simulink model "px4_6dof_quadrotor_bus"  (R2021b)
settings: Solver=VariableStepAuto  StartTime=0.0  StopTime=10.0  FixedStep=plant.motor.dynamic_time_sample/10  RelTol=1e-3
undefined symbols (not defined in the file or in its folder): angular_rate, ax, ay, az, body, controller, DiscIntNeverNeededParam, dphi, dpsi, dtheta, lag, land_detector, lead, magnitude, ned, notch, phi, pitch, plant, psi, rad, roll, s, theta, thrust, vx, vy, vz, w1, w2, w3, w4, x, y, yaw, z
libraries: cstblocks x33, aerolibconvert2 x4, simulink_extras x3, simulink x3, sharedtransform x1
(part 2 of 2)

== system px4_6dof_quadrotor_bus/plant/control2motors/Plant1/Subsystem ==
  In1 : Inport
  Discrete-Time Integrator : DiscreteIntegrator  SampleTime=-1  ICPrevOutput=DiscIntNeverNeededParam  ICPrevScaledInput=DiscIntNeverNeededParam
  Gain : Gain  Gain=plant.motor.r
  Gain1 : Gain  Gain=1/plant.motor.l
  Sum : Sum  Inputs=|+-
  Im : Outport
  wires:
  Gain/1 -> Sum/2
  Gain1/1 -> Discrete-Time Integrator/1
  Discrete-Time Integrator/1 -> Im/1, Gain/1
  Sum/1 -> Gain1/1
  In1/1 -> Sum/1

== system px4_6dof_quadrotor_bus/plant/control2motors/Plant1/Subsystem1 ==
  In1 : Inport
  Discrete-Time Integrator : DiscreteIntegrator  SampleTime=plant.motor.electric_time_sample  ICPrevOutput=DiscIntNeverNeededParam  ICPrevScaledInput=DiscIntNeverNeededParam
  Gain : Gain  Gain=1/plant.motor.j_m
  Out1 : Outport
  wires:
  Gain/1 -> Out1/1
  Discrete-Time Integrator/1 -> Gain/1
  In1/1 -> Discrete-Time Integrator/1

== system px4_6dof_quadrotor_bus/plant/control2motors/Plant1/Subsystem2 ==
  In1 : Inport
  Discrete-Time Integrator : DiscreteIntegrator  SampleTime=plant.motor.electric_time_sample  ICPrevOutput=DiscIntNeverNeededParam  ICPrevScaledInput=DiscIntNeverNeededParam
  Gain : Gain  Gain=1/plant.motor.j_l
  Out1 : Outport
  wires:
  Gain/1 -> Out1/1
  In1/1 -> Discrete-Time Integrator/1
  Discrete-Time Integrator/1 -> Gain/1

== system px4_6dof_quadrotor_bus/plant/control2motors/Plant1/Subsystem3 ==
  dvel : Inport
  Add : Sum
  Discrete-Time Integrator : DiscreteIntegrator  SampleTime=plant.motor.electric_time_sample  ICPrevOutput=DiscIntNeverNeededParam  ICPrevScaledInput=DiscIntNeverNeededParam
  Gain2 : Gain  Gain=plant.motor.k_v
  Gain5 : Gain  Gain=plant.motor.k_k
  Tload : Outport
  wires:
  Add/1 -> Tload/1
  Gain2/1 -> Add/1
  Gain5/1 -> Add/2
  dvel/1 -> Discrete-Time Integrator/1, Gain2/1
  Discrete-Time Integrator/1 -> Gain5/1

== system px4_6dof_quadrotor_bus/plant/control2motors/Plant2/Subsystem ==
  In1 : Inport
  Discrete-Time Integrator : DiscreteIntegrator  SampleTime=-1  ICPrevOutput=DiscIntNeverNeededParam  ICPrevScaledInput=DiscIntNeverNeededParam
  Gain : Gain  Gain=plant.motor.r
  Gain1 : Gain  Gain=1/plant.motor.l
  Sum : Sum  Inputs=|+-
  Im : Outport
  wires:
  Gain/1 -> Sum/2
  Gain1/1 -> Discrete-Time Integrator/1
  Discrete-Time Integrator/1 -> Im/1, Gain/1
  Sum/1 -> Gain1/1
  In1/1 -> Sum/1

== system px4_6dof_quadrotor_bus/plant/control2motors/Plant2/Subsystem1 ==
  In1 : Inport
  Discrete-Time Integrator : DiscreteIntegrator  SampleTime=plant.motor.electric_time_sample  ICPrevOutput=DiscIntNeverNeededParam  ICPrevScaledInput=DiscIntNeverNeededParam
  Gain : Gain  Gain=1/plant.motor.j_m
  Out1 : Outport
  wires:
  Gain/1 -> Out1/1
  Discrete-Time Integrator/1 -> Gain/1
  In1/1 -> Discrete-Time Integrator/1

== system px4_6dof_quadrotor_bus/plant/control2motors/Plant2/Subsystem2 ==
  In1 : Inport
  Discrete-Time Integrator : DiscreteIntegrator  SampleTime=plant.motor.electric_time_sample  ICPrevOutput=DiscIntNeverNeededParam  ICPrevScaledInput=DiscIntNeverNeededParam
  Gain : Gain  Gain=1/plant.motor.j_l
  Out1 : Outport
  wires:
  Gain/1 -> Out1/1
  In1/1 -> Discrete-Time Integrator/1
  Discrete-Time Integrator/1 -> Gain/1

== system px4_6dof_quadrotor_bus/plant/control2motors/Plant2/Subsystem3 ==
  dvel : Inport
  Add : Sum
  Discrete-Time Integrator : DiscreteIntegrator  SampleTime=plant.motor.electric_time_sample  ICPrevOutput=DiscIntNeverNeededParam  ICPrevScaledInput=DiscIntNeverNeededParam
  Gain2 : Gain  Gain=plant.motor.k_v
  Gain5 : Gain  Gain=plant.motor.k_k
  Tload : Outport
  wires:
  Add/1 -> Tload/1
  Gain2/1 -> Add/1
  Gain5/1 -> Add/2
  dvel/1 -> Discrete-Time Integrator/1, Gain2/1
  Discrete-Time Integrator/1 -> Gain5/1

== system px4_6dof_quadrotor_bus/plant/control2motors/Plant3/Subsystem ==
  In1 : Inport
  Discrete-Time Integrator : DiscreteIntegrator  SampleTime=-1  ICPrevOutput=DiscIntNeverNeededParam  ICPrevScaledInput=DiscIntNeverNeededParam
  Gain : Gain  Gain=plant.motor.r
  Gain1 : Gain  Gain=1/plant.motor.l
  Sum : Sum  Inputs=|+-
  Im : Outport
  wires:
  Gain/1 -> Sum/2
  Gain1/1 -> Discrete-Time Integrator/1
  Discrete-Time Integrator/1 -> Im/1, Gain/1
  Sum/1 -> Gain1/1
  In1/1 -> Sum/1

== system px4_6dof_quadrotor_bus/plant/control2motors/Plant3/Subsystem1 ==
  In1 : Inport
  Discrete-Time Integrator : DiscreteIntegrator  SampleTime=plant.motor.electric_time_sample  ICPrevOutput=DiscIntNeverNeededParam  ICPrevScaledInput=DiscIntNeverNeededParam
  Gain : Gain  Gain=1/plant.motor.j_m
  Out1 : Outport
  wires:
  Gain/1 -> Out1/1
  Discrete-Time Integrator/1 -> Gain/1
  In1/1 -> Discrete-Time Integrator/1

== system px4_6dof_quadrotor_bus/plant/control2motors/Plant3/Subsystem2 ==
  In1 : Inport
  Discrete-Time Integrator : DiscreteIntegrator  SampleTime=plant.motor.electric_time_sample  ICPrevOutput=DiscIntNeverNeededParam  ICPrevScaledInput=DiscIntNeverNeededParam
  Gain : Gain  Gain=1/plant.motor.j_l
  Out1 : Outport
  wires:
  Gain/1 -> Out1/1
  In1/1 -> Discrete-Time Integrator/1
  Discrete-Time Integrator/1 -> Gain/1

== system px4_6dof_quadrotor_bus/plant/control2motors/Plant3/Subsystem3 ==
  dvel : Inport
  Add : Sum
  Discrete-Time Integrator : DiscreteIntegrator  SampleTime=plant.motor.electric_time_sample  ICPrevOutput=DiscIntNeverNeededParam  ICPrevScaledInput=DiscIntNeverNeededParam
  Gain2 : Gain  Gain=plant.motor.k_v
  Gain5 : Gain  Gain=plant.motor.k_k
  Tload : Outport
  wires:
  Add/1 -> Tload/1
  Gain2/1 -> Add/1
  Gain5/1 -> Add/2
  dvel/1 -> Discrete-Time Integrator/1, Gain2/1
  Discrete-Time Integrator/1 -> Gain5/1

== system px4_6dof_quadrotor_bus/plant/control2motors/Velocity Controller/Lag1 ==
  In1 : Inport
  LTI System : cstblocks/LTI System  sys=lag(Freq,Beta)  IC=[]
  Out1 : Outport
  wires:
  In1/1 -> LTI System/1
  LTI System/1 -> Out1/1

== system px4_6dof_quadrotor_bus/plant/control2motors/Velocity Controller/Notch ==
  In1 : Inport
  LTI System : cstblocks/LTI System  sys=notch(wn,wd,zn,zd)  IC=[]
  Out1 : Outport
  wires:
  LTI System/1 -> Out1/1
  In1/1 -> LTI System/1

== system px4_6dof_quadrotor_bus/plant/control2motors/Velocity Controller/Subsystem1 ==
  In1 : Inport
  LTI System : cstblocks/LTI System  sys=lead(Phase,Freq)  IC=[]
  Out1 : Outport
  wires:
  In1/1 -> LTI System/1
  LTI System/1 -> Out1/1

== system px4_6dof_quadrotor_bus/plant/control2motors/Velocity Controller1/Lag1 ==
  In1 : Inport
  LTI System : cstblocks/LTI System  sys=lag(Freq,Beta)  IC=[]
  Out1 : Outport
  wires:
  In1/1 -> LTI System/1
  LTI System/1 -> Out1/1

== system px4_6dof_quadrotor_bus/plant/control2motors/Velocity Controller1/Notch ==
  In1 : Inport
  LTI System : cstblocks/LTI System  sys=notch(wn,wd,zn,zd)  IC=[]
  Out1 : Outport
  wires:
  LTI System/1 -> Out1/1
  In1/1 -> LTI System/1

== system px4_6dof_quadrotor_bus/plant/control2motors/Velocity Controller1/Subsystem1 ==
  In1 : Inport
  LTI System : cstblocks/LTI System  sys=lead(Phase,Freq)  IC=[]
  Out1 : Outport
  wires:
  In1/1 -> LTI System/1
  LTI System/1 -> Out1/1

== system px4_6dof_quadrotor_bus/plant/control2motors/Velocity Controller2/Lag1 ==
  In1 : Inport
  LTI System : cstblocks/LTI System  sys=lag(Freq,Beta)  IC=[]
  Out1 : Outport
  wires:
  In1/1 -> LTI System/1
  LTI System/1 -> Out1/1

== system px4_6dof_quadrotor_bus/plant/control2motors/Velocity Controller2/Notch ==
  In1 : Inport
  LTI System : cstblocks/LTI System  sys=notch(wn,wd,zn,zd)  IC=[]
  Out1 : Outport
  wires:
  LTI System/1 -> Out1/1
  In1/1 -> LTI System/1

== system px4_6dof_quadrotor_bus/plant/control2motors/Velocity Controller2/Subsystem1 ==
  In1 : Inport
  LTI System : cstblocks/LTI System  sys=lead(Phase,Freq)  IC=[]
  Out1 : Outport
  wires:
  In1/1 -> LTI System/1
  LTI System/1 -> Out1/1

== system px4_6dof_quadrotor_bus/plant/control2motors/Velocity Controller3/Lag1 ==
  In1 : Inport
  LTI System : cstblocks/LTI System  sys=lag(Freq,Beta)  IC=[]
  Out1 : Outport
  wires:
  In1/1 -> LTI System/1
  LTI System/1 -> Out1/1

== system px4_6dof_quadrotor_bus/plant/control2motors/Velocity Controller3/Notch ==
  In1 : Inport
  LTI System : cstblocks/LTI System  sys=notch(wn,wd,zn,zd)  IC=[]
  Out1 : Outport
  wires:
  LTI System/1 -> Out1/1
  In1/1 -> LTI System/1

== system px4_6dof_quadrotor_bus/plant/control2motors/Velocity Controller3/Subsystem1 ==
  In1 : Inport
  LTI System : cstblocks/LTI System  sys=lead(Phase,Freq)  IC=[]
  Out1 : Outport
  wires:
  In1/1 -> LTI System/1
  LTI System/1 -> Out1/1

== matlab function px4_6dof_quadrotor_bus/plant/body2ned/Second Law in Z/LandDetector ==
  settings: updateMethod=DISCRETE
  data: ddz_raw input; ddz output; z input; land_detector output
function [ddz, land_detector] = fcn(ddz_raw,z)

persistent takeOff

if isempty(takeOff)
    takeOff = false;
end

if ~takeOff && z < -0.2
    takeOff = true;

end

if takeOff && z > -0.01 
    ddz = 0.0;
    land_detector = true;
else
    ddz = ddz_raw;
    land_detector = false;
end

== matlab function px4_6dof_quadrotor_bus/mixer/MATLAB Function ==
  data: mat input; y output; vect input
function y = fcn(mat,vect)
y = mat\vect;

== matlab function px4_6dof_quadrotor_bus/plant/body2ned/stop_integrate_velocity ==
  data: vz_raw input; v output; land_detector input
function v = fcn(vz_raw, land_detector)

if land_detector
    v = 0.0;
else
    v = vz_raw;
end
